simulink model "Exp_3_batch_12_simulation2"  (R2020a)
settings: Solver=VariableStepAuto  StartTime=0.0  StopTime=20  RelTol=1e-3
settings Model: Creator=sundaram bhupathi  LastModifiedBy=sundaram bhupathi

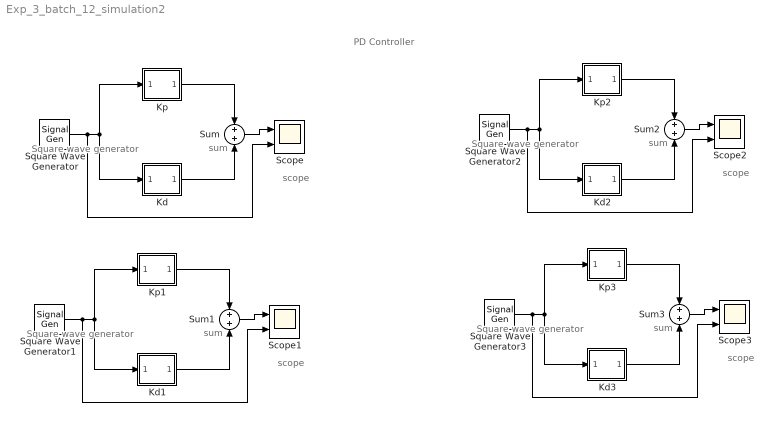
== system Exp_3_batch_12_simulation2 ==
  note: PD Controller
  note: scope
  note: Square wave generator
  note: sum
  note: sum
  note: Square wave generator
  note: scope
  note: sum
  note: Square wave generator
  note: scope
  note: sum
  note: Square wave generator
  note: scope
  Kd : Subsystem
  Kd1 : Subsystem
  Kd2 : Subsystem
  Kd3 : Subsystem
  Kp : Subsystem
  Kp1 : Subsystem
  Kp2 : Subsystem
  Kp3 : Subsystem
  Scope{,1..3} (4 alike) : Scope  NumInputPorts=2
  Square Wave Generator{,1..3} (4 alike) : SignalGenerator  WaveForm=square  Amplitude=10  Units=rad/sec
  Sum{,1..3} (4 alike) : Sum  InputSameDT=on  SaturateOnIntegerOverflow=on  OutDataTypeStr=Inherit: Same as first input
  wires:
  Kd/1(Out1) -> Sum/2
  Square Wave Generator/1 -> Scope/2, Kd/1(In1), Kp/1(In1)
  Kp/1(Out1) -> Sum/1
  Sum/1 -> Scope/1
  Kp1/1(Out1) -> Sum1/1
  Square Wave Generator1/1 -> Scope1/2, Kd1/1(In1), Kp1/1(In1)
  Sum1/1 -> Scope1/1
  Kd1/1(Out1) -> Sum1/2
  Kp2/1(Out1) -> Sum2/1
  Square Wave Generator2/1 -> Scope2/2, Kd2/1(In1), Kp2/1(In1)
  Sum2/1 -> Scope2/1
  Kd2/1(Out1) -> Sum2/2
  Kp3/1(Out1) -> Sum3/1
  Square Wave Generator3/1 -> Scope3/2, Kd3/1(In1), Kp3/1(In1)
  Sum3/1 -> Scope3/1
  Kd3/1(Out1) -> Sum3/2

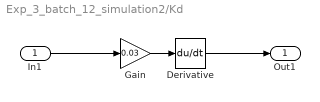
== system Exp_3_batch_12_simulation2/Kd ==
  In1 : Inport
  Derivative : Derivative
  Gain : Gain  Gain=0.03
  Out1 : Outport
  wires:
  In1/1 -> Gain/1
  Gain/1 -> Derivative/1
  Derivative/1 -> Out1/1

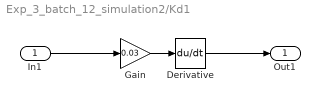
== system Exp_3_batch_12_simulation2/Kd1 ==
  In1 : Inport
  Derivative : Derivative
  Gain : Gain  Gain=0.03
  Out1 : Outport
  wires:
  In1/1 -> Gain/1
  Gain/1 -> Derivative/1
  Derivative/1 -> Out1/1

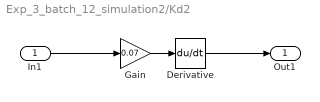
== system Exp_3_batch_12_simulation2/Kd2 ==
  In1 : Inport
  Derivative : Derivative
  Gain : Gain  Gain=0.07
  Out1 : Outport
  wires:
  In1/1 -> Gain/1
  Gain/1 -> Derivative/1
  Derivative/1 -> Out1/1

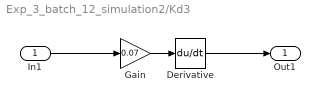
== system Exp_3_batch_12_simulation2/Kd3 ==
  In1 : Inport
  Derivative : Derivative
  Gain : Gain  Gain=0.07
  Out1 : Outport
  wires:
  In1/1 -> Gain/1
  Gain/1 -> Derivative/1
  Derivative/1 -> Out1/1

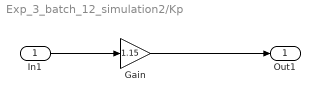
== system Exp_3_batch_12_simulation2/Kp ==
  In1 : Inport
  Gain : Gain  Gain=1.15
  Out1 : Outport
  wires:
  In1/1 -> Gain/1
  Gain/1 -> Out1/1

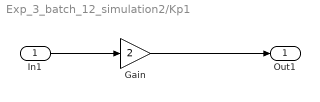
== system Exp_3_batch_12_simulation2/Kp1 ==
  In1 : Inport
  Gain : Gain  Gain=2
  Out1 : Outport
  wires:
  In1/1 -> Gain/1
  Gain/1 -> Out1/1

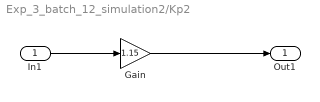
== system Exp_3_batch_12_simulation2/Kp2 ==
  In1 : Inport
  Gain : Gain  Gain=1.15
  Out1 : Outport
  wires:
  In1/1 -> Gain/1
  Gain/1 -> Out1/1

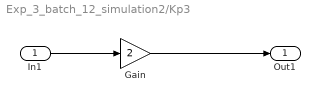
== system Exp_3_batch_12_simulation2/Kp3 ==
  In1 : Inport
  Gain : Gain  Gain=2
  Out1 : Outport
  wires:
  In1/1 -> Gain/1
  Gain/1 -> Out1/1
